simulink model "ScriptDemo"  (R2022b)
settings: configuration reference "TmVcThermal_Configuration_sub" (kept outside this file)
undefined symbols (not defined in the file or in its folder): aaaa, bbbb, cTmComprCtrl_D_u8HvacFlowTable_db, cTmComprCtrl_D_u8HvacFlowTable_sw, cTmComprCtrl_n_i16ChillCmpIMax, cTmComprCtrl_n_i16ChillCmpIMin, cTmComprCtrl_n_i16ChillCmpIMin666, cTmComprCtrl_n_i16ChillCmpPMax, cTmComprCtrl_n_i16ChillCmpPMin, cTmComprCtrl_n_i16CmpChillCoolRpmKiMax, cTmComprCtrl_n_i16CmpChillCoolRpmKiMin, cTmComprCtrl_n_i16CmpChillCoolRpmKpMax, cTmComprCtrl_n_i16CmpChillCoolRpmKpMin, cTmComprCtrl_n_i16CmpCoolRpmKiMax, cTmComprCtrl_n_i16CmpCoolRpmKiMin, cTmComprCtrl_n_i16CmpCoolRpmKpMax, cTmComprCtrl_n_i16CmpCoolRpmKpMin, cTmComprCtrl_n_i16SM4CmpHeatKiMax, cTmComprCtrl_n_i16SM4CmpHeatKiMin, cTmComprCtrl_n_i16SM4CmpHeatKpMax, cTmComprCtrl_n_i16SM4CmpHeatKpMin, cTmComprCtrl_n_i16SM5CmpHeatKiMax, cTmComprCtrl_n_i16SM5CmpHeatKiMin, cTmComprCtrl_n_i16SM5CmpHeatKpMax, cTmComprCtrl_n_i16SM5CmpHeatKpMin, cTmComprCtrl_n_i16SM6CmpHeatKiMax, cTmComprCtrl_n_i16SM6CmpHeatKiMin, cTmComprCtrl_n_i16SM6CmpHeatKpMax, cTmComprCtrl_n_i16SM6CmpHeatKpMin, cTmComprCtrl_n_u16CmpMaxSpdFanFltLimt, cTmComprCtrl_n_u16CmpMaxSpdLoSidePFltLimt, cTmComprCtrl_n_u16CmpMaxSpdSensorFltLimt, cTmComprCtrl_n_u16CompMinRpm, cTmComprCtrl_n_u16CompRpmIncThres, cTmComprCtrl_t_u16BattCooltFFPeriod, cTmComprCtrl_t_u16BattCooltPIPeriod, cTmComprCtrl_t_u16CmpCoolFFPeriod, cTmComprCtrl_t_u16CmpCoolPIPeriod, cTmComprCtrl_t_u16CoolCmpChillFFPeriod, cTmComprCtrl_t_u16CoolCmpChillPIPeriod, cTmComprCtrl_t_u16SM4CmpHeatFFPeriod, cTmComprCtrl_t_u16SM4CmpHeatPIPeriod, cTmComprCtrl_t_u16SM5CmpHeatFFPeriod, cTmComprCtrl_t_u16SM5CmpHeatPIPeriod, cTmComprCtrl_t_u16SM6CmpHeatFFPeriod, cTmComprCtrl_t_u16SM6CmpHeatPIPeriod, cTmComprCtrl_Te_EvapClearInteg, cTmComprCtrl_Te_i16HpReqTempSaturoffset, cTmComprCtrl_Te_i16SatLpReplaceDiff, cTmComprCtrl_Te_i16SM3BatDiffStartEvapDecOffset, cTmComprCtrl_Te_i16SM3EvapLo, cTmComprCtrl_Te_i16SM3TBatDiffEntEvapDecOffset, cTmComprCtrl_Te_i16SM3TBatDiffEntEvapDecOffsetQuit, cTmComprCtrl_Te_s32ErrCmpChillPIContinueCoolH, cTmComprCtrl_Te_s32ErrCmpChillPIContinueCoolL, cTmComprCtrl_Te_s32ErrCmpPIContinueChillH, cTmComprCtrl_Te_s32ErrCmpPIContinueChillL, cTmComprCtrl_Te_s32ErrCmpPIContinueCoolH, cTmComprCtrl_Te_s32ErrCmpPIContinueCoolL, cTmComprCtrl_Te_s32ErrCmpPIContinueHeatH ... (+398)
libraries: simulink x846, PCMULib x711, simulink_need_slupdate x4
(part 10 of 49)

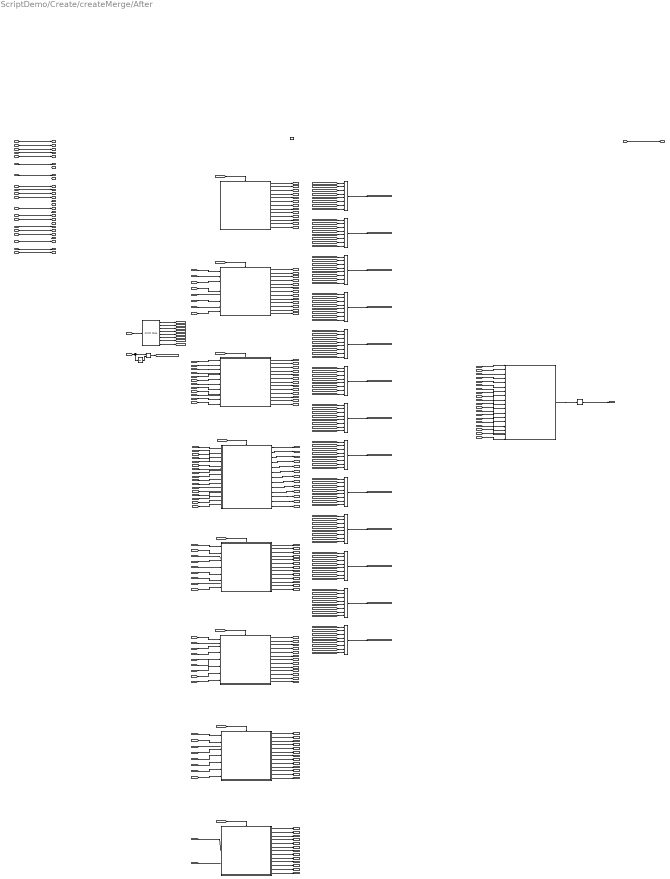
== system ScriptDemo/Create/createMerge/After ==
  note: % 目的: 对当前路径下的，使能子系统或switch case输出的信号，自动生成Merge
      | createMerge( ...
      | 'sigList' , ...
      | { 'rTmComprCtrl_Te_s32LowErrStop' , 'rTmComprCtrl_Te_s32TempError' , ...
      | 'rTmComprCtrl_Te_s32UpErrStop' , 'rTmComprCtrl_n_u16ComprRpmFF' , ...
      | 'rTmComprCtrl_n_u16ComprRpmKi' , 'rTmComprCtrl_n_u16ComprRpmKp' , ...
      | 'rTmComprCtrl_n_u16DisOverrideValue' , 'rTmComprCtrl_n_i16KiLowLimit' , ...
      | 'rTmComprCtrl_n_i16KiUpLimit' , 'rTmComprCtrl_n_i16KpLowLimit' , ...
      | 'rTmComprCtrl_n_i16KpUpLimit' , 'rTmComprCtrl_t_u16PIPeriod' , ...
      | 'xTmComprCtrl_B_Enable' ...
      | }, ...
      | 'resovleSig' ,true)
      |
      | %% 输入参数处理
      | p = inputParser; % 函数的输入解析器
      | addParameter(p, 'sigList' , ...
      | { 'rTmComprCtrl_Te_s32TempError' , 'rTmComprCtrl_n_u16ComprRpmFF' , ...
      | 'rTmComprCtrl_n_u16ComprRpmKp' , 'rTmComprCtrl_n_u16ComprRpmKi' , ...
      | 'rTmComprCtrl_Te_s32UpErrStop' , 'rTmComprCtrl_Te_s32LowErrStop' , ...
      | 'rTmComprCtrl_n_u16KpUpLimit' , 'rTmComprCtrl_n_u16KpLowLimit' , ...
      | 'rTmComprCtrl_n_u16KiUpLimit' , 'rTmComprCtrl_n_u16KiLowLimit' , ...
      | 'rTmComprCtrl_n_u16DisOverrideValue' , 'rTmComprCtrl_t_u8PIPeriod' , ...
      | 'rTmComprCtrl_B_Enable'
      | } ...
      | ); % 设置变量名
      | addParameter(p, 'resovleSig' ,true); % 是否需要解析merge的信号
  sTmComprCtrl_D_u8HvacFlowLevel : Inport  OutDataTypeStr=uint8
  sTmSigProces_Te_s32EvapFanReqRamp : Inport  Port=2  OutDataTypeStr=single
  sTmDiag_D_u8TeEvapFltSt : Inport  Port=3  OutDataTypeStr=uint8
  sTmIn_D_u8DCChrgSt : Inport  Port=4  OutDataTypeStr=uint8
  sTmIn_D_u8HeatPump : Inport  Port=5  OutDataTypeStr=uint8
  sTmIn_Te_s32BattHv : Inport  Port=6  OutDataTypeStr=single
  sTmIn_X_s32ClimtRcirc : Inport  Port=7  OutDataTypeStr=single
  sTmSigProces_D_u8BattThermReq : Inport  Port=8  OutDataTypeStr=uint8
  sTmSigProces_D_u8HvBattCoolgReq : Inport  Port=9  OutDataTypeStr=uint8
  sTmSigProces_Te_s32EvapFanFilter : Inport  Port=10  OutDataTypeStr=single
  sTmSigProces_Te_s32HeatrAirTReqRamp : Inport  Port=11  OutDataTypeStr=single
  sTmSigProces_Te_s32HvacHexAirTFilter : Inport  Port=12  OutDataTypeStr=single
  sTmSigProces_Te_s32SatHp : Inport  Port=13  OutDataTypeStr=single
  sTmSigProces_Te_s32SatLp : Inport  Port=14  OutDataTypeStr=single
  xTmComprCtrl_B_CompOnReqCompOn : Inport  Port=15  OutDataTypeStr=boolean
  xTmComprCtrl_B_ReduceRpm : Inport  Port=16  OutDataTypeStr=boolean
  yTmHvchCtrl_B_HpcPtcEnad : Inport  Port=17  OutDataTypeStr=boolean
  yTmRefriModeMgr_B_CoolOCRMode : Inport  Port=18  OutDataTypeStr=boolean
  sTmSigProces_Pw_i16ReqPwrForCool : Inport  Port=19  OutDataTypeStr=int16
  yTmRefriModeMgr_B_HeatModeInCycle : Inport  Port=20  OutDataTypeStr=boolean
  Enable : EnablePort
  ID29332_RpmPI : Subsystem
  Merge{,1..12} (13 alike) : Merge  Inputs=8
  Relational Operator : RelationalOperator  Operator=~=  OutDataTypeStr=boolean  RndMeth=Simplest  InputSameDT=off
  SM0 : Subsystem
  SM1SM21 : Subsystem
  SM2SM22 : Subsystem
  SM3SM23 : Subsystem
  SM4 : Subsystem
  SM5 : Subsystem
  SM6 : Subsystem
  SM7 : Subsystem
  Signal Conversion : SignalConversion  OverrideOpt=off
  Switch Case : SwitchCase  CaseConditions={0,[1,21],[2,22],[3,23],4,5,6,7}  ShowDefaultCase=off
  Unit Delay : UnitDelay  SampleTime=-1  HasFrameUpgradeWarning=on
  sTmComprCtrl_n_u16CompRpmReqNorm : Outport  OutDataTypeStr=uint16
  wires:
  [yTmRefriModeMgr_B_CoolOCRMode] -> SM2SM22/9(yTmRefriModeMgr_B_CoolOCRMode)
  ? -> [sTmIn_Te_s32HvBattCooltTReq]
  [sTmSigProces_D_u8BattThermReq] -> SM3SM23/8(sTmSigProces_D_u8BattThermReq)
  [sTmSigProces_Te_s32TempInlet] -> ?
  ? -> [yTmRefriModeMgr_B_CoolModeInCycle]
  [sTmSigProces_Te_s32SatHp] -> SM5/4(sTmSigProces_Te_s32SatHp)
  [sTmRefriModeMgr_D_u8HPCurMode] -> ?
  [yTmRefriModeMgr_B_HeatModeInCycle] -> SM4/7(yTmRefriModeMgr_B_HeatModeInCycle)
  [xTmComprCtrl_B_ModeChanged] -> SM3SM23/13(xTmComprCtrl_B_ModeChanged)
  [yTmRefriModeMgr_B_HeatModeInCycle] -> SM6/7(yTmRefriModeMgr_B_HeatModeInCycle)
  [yTmRefriModeMgr_B_CoolModeInCycle] -> ?
  [SM5] -> SM5/Action
  sTmSigProces_Te_s32SatLp/1 -> [sTmSigProces_Te_s32SatLp]
  sTmIn_X_s32ClimtRcirc/1 -> [sTmIn_X_s32ClimtRcirc]
  yTmRefriModeMgr_B_HeatModeInCycle/1 -> [yTmRefriModeMgr_B_HeatModeInCycle]
  yTmRefriModeMgr_B_CoolOCRMode/1 -> [yTmRefriModeMgr_B_CoolOCRMode]
  [yTmRefriModeMgr_B_HeatModeInCycle] -> ID29332_RpmPI/18(yTmRefriModeMgr_B_HeatModeInCycle)
  yTmHvchCtrl_B_HpcPtcEnad/1 -> [yTmHvchCtrl_B_HpcPtcEnad]
  [sTmSigProces_Te_s32EvapFanFilter] -> ID29332_RpmPI/17(sTmSigProces_Te_s32EvapFanFilter)
  [sTmSigProces_D_u8HvBattCoolgReq] -> SM3SM23/9(sTmSigProces_D_u8HvBattCoolgReq)
  [sTmSigProces_Te_s32HvacHexAirTFilter] -> SM5/3(sTmSigProces_Te_s32HvacHexAirTFilter)
  ? -> [sTmSigProces_Te_s32HvBattCooltTFilter]
  [yTmRefriModeMgr_B_CoolOCRMode] -> SM3SM23/14(yTmRefriModeMgr_B_CoolOCRMode)
  [yTmHvchCtrl_B_HpcPtcEnad] -> SM5/7(yTmHvchCtrl_B_HpcPtcEnad)
  [sTmComprCtrl_D_u8HvacFlowLevel] -> SM5/5(sTmComprCtrl_D_u8HvacFlowLevel)
  sTmSigProces_D_u8HvBattCoolgReq/1 -> [sTmSigProces_D_u8HvBattCoolgReq]
  [xTmComprCtrl_B_ReduceRpm] -> ID29332_RpmPI/16(xTmComprCtrl_B_ReduceRpm)
  ? -> [sTmSigProces_Te_s32HvBattCooltTOutFilter]
  sTmSigProces_Pw_i16ReqPwrForCool/1 -> [sTmSigProces_Pw_i16ReqPwrForCool]
  [sTmSigProces_Te_s32TAmb] -> ?
  [sTmIn_Te_s32BattHv] -> SM3SM23/5(sTmIn_Te_s32BattHv)
  [sTmComprCtrl_D_u8HvacFlowLevel] -> SM6/4(sTmComprCtrl_D_u8HvacFlowLevel)
  Switch Case/7 -> [SM6]
  Switch Case/5 -> [SM4]
  ? -> [sTmSigProces_Te_s32TempInlet]
  [xTmComprCtrl_B_CompOnReqCompOn] -> SM5/6(xTmComprCtrl_B_CompOnReqCompOn)
  [rTmComprCtrl_n_u16ComprRpmKp] -> ID29332_RpmPI/6(rTmComprCtrl_n_u16ComprRpmKp)
  [SM0] -> SM0/Action
  xTmComprCtrl_B_ReduceRpm/1 -> [xTmComprCtrl_B_ReduceRpm]
  [sTmSigProces_Te_s32HeatrAirTReqRamp] -> SM6/1(sTmSigProces_Te_s32HeatrAirTReqRamp)
  Relational Operator/1 -> [xTmComprCtrl_B_ModeChanged]
  [xTmComprCtrl_B_CompOnReqCompOn] -> SM3SM23/12(xTmComprCtrl_B_CompOnReqCompOn)
  sTmSigProces_Te_s32EvapFanFilter/1 -> [sTmSigProces_Te_s32EvapFanFilter]
  [xTmComprCtrl_B_CompOnReqCompOn] -> SM6/5(xTmComprCtrl_B_CompOnReqCompOn)
  [sTmSigProces_Te_s32HvacHexAirTFilter] -> SM4/2(sTmSigProces_Te_s32HvacHexAirTFilter)
  [sTmSigProces_Te_s32HvBattCooltTFilter] -> ?
  [yTmHvchCtrl_B_HpcPtcEnad] -> SM6/6(yTmHvchCtrl_B_HpcPtcEnad)
  [rTmComprCtrl_Te_s32TempError] -> ID29332_RpmPI/2(rTmComprCtrl_Te_s32TempError)
  [sTmSigProces_Te_s32SatHp] -> SM6/3(sTmSigProces_Te_s32SatHp)
  [sTmIn_D_u8DCChrgSt] -> SM1SM21/1(sTmIn_D_u8DCChrgSt)
  [SM6] -> SM6/Action
  [sTmIn_D_u8DCChrgSt] -> SM3SM23/3(sTmIn_D_u8DCChrgSt)
  [xTmComprCtrl_B_CompOnReqCompOn] -> SM4/5(xTmComprCtrl_B_CompOnReqCompOn)
  [sTmSigProces_Te_s32HvBattCooltTFilter] -> ?
  Switch Case/4 -> [SM3_SM23]
  [rTmComprCtrl_n_u16ComprRpmFF] -> ID29332_RpmPI/4(rTmComprCtrl_n_u16ComprRpmFF)
  [xTmComprCtrl_B_Enable] -> ID29332_RpmPI/14(xTmComprCtrl_B_Enable)
  [sTmSigProces_Te_s32TAmb] -> ?
  [rTmComprCtrl_n_i16KpLowLimit] -> ID29332_RpmPI/10(rTmComprCtrl_n_i16KpLowLimit)
  [rTmComprCtrl_n_u16DisOverrideValue] -> ID29332_RpmPI/7(rTmComprCtrl_n_u16DisOverrideValue)
  xTmComprCtrl_B_CompOnReqCompOn/1 -> [xTmComprCtrl_B_CompOnReqCompOn]
  [rTmComprCtrl_n_u16ComprRpmKi] -> ID29332_RpmPI/5(rTmComprCtrl_n_u16ComprRpmKi)
  [rTmComprCtrl_n_i16KiLowLimit] -> ID29332_RpmPI/8(rTmComprCtrl_n_i16KiLowLimit)
  [xTmComprCtrl_B_ModeChanged] -> ID29332_RpmPI/15(xTmComprCtrl_B_ModeChanged)
  [sTmSigProces_Te_s32HvBattCooltTFilter] -> ?
  [sTmSigProces_Te_s32TempInlet] -> ?
  [sTmIn_Te_s32HvBattCooltTReq] -> ?
  Unit Delay/1 -> Relational Operator/2
  [SM2_SM22] -> SM2SM22/Action
  [sTmIn_D_u8HeatPump] -> SM3SM23/4(sTmIn_D_u8HeatPump)
  [sTmSigProces_Te_s32TAmb] -> ?
  [sTmRefriModeMgr_D_u8HPCurMode] -> Switch Case/1
  [sTmSigProces_Te_s32HeatrAirTReqRamp] -> SM5/2(sTmSigProces_Te_s32HeatrAirTReqRamp)
  [rTmComprCtrl_n_i16KpUpLimit] -> ID29332_RpmPI/11(rTmComprCtrl_n_i16KpUpLimit)
  [sTmComprCtrl_D_u8HvacFlowLevel] -> SM3SM23/7(sTmComprCtrl_D_u8HvacFlowLevel)
  [rTmComprCtrl_Te_s32LowErrStop] -> ID29332_RpmPI/1(rTmComprCtrl_Te_s32LowErrStop)
  [sTmSigProces_Te_s32EvapFanReqRamp] -> SM3SM23/1(sTmSigProces_Te_s32EvapFanReqRamp)
  [sTmSigProces_D_u8HvBattCoolgReq] -> SM1SM21/3(sTmSigProces_D_u8HvBattCoolgReq)
  [sTmComprCtrl_D_u8HvacFlowLevel] -> SM2SM22/5(sTmComprCtrl_D_u8HvacFlowLevel)
  Switch Case/8 -> [SM7]
  [sTmSigProces_Te_s32EvapFanReqRamp] -> SM2SM22/1(sTmSigProces_Te_s32EvapFanReqRamp)
  [sTmRefriModeMgr_D_u8HPCurMode] -> Unit Delay/1, Relational Operator/1
  [SM4] -> SM4/Action
  [sTmSigProces_Te_s32SatLp] -> SM2SM22/7(sTmSigProces_Te_s32SatLp)
  [sTmIn_D_u8HeatPump] -> SM2SM22/3(sTmIn_D_u8HeatPump)
  [sTmSigProces_Te_s32SatLp] -> SM3SM23/11(sTmSigProces_Te_s32SatLp)
  [sTmSigProces_Te_s32EvapFanFilter] -> SM2SM22/6(sTmSigProces_Te_s32EvapFanFilter)
  [sTmSigProces_Te_s32SatHp] -> SM4/3(sTmSigProces_Te_s32SatHp)
  [sTmSigProces_Pw_i16ReqPwrForCool] -> SM2SM22/10(sTmSigProces_Pw_i16ReqPwrForCool)
  [SM7] -> SM7/Action
  ? -> [sTmSigProces_Te_s32TAmb]
  [sTmSigProces_Te_s32TempInlet] -> ?
  [sTmDiag_D_u8TeEvapFltSt] -> SM3SM23/2(sTmDiag_D_u8TeEvapFltSt)
  [sTmSigProces_Te_s32HvacHexAirTFilter] -> SM6/2(sTmSigProces_Te_s32HvacHexAirTFilter)
  [sTmSigProces_Te_s32TAmb] -> ?
  [sTmIn_D_u8HeatPump] -> SM1SM21/5(sTmIn_D_u8HeatPump)
  [yTmRefriModeMgr_B_CoolModeInCycle] -> ?
  [sTmIn_X_s32ClimtRcirc] -> SM2SM22/4(sTmIn_X_s32ClimtRcirc)
  [SM1_SM21] -> SM1SM21/Action
  [sTmIn_X_s32ClimtRcirc] -> SM3SM23/6(sTmIn_X_s32ClimtRcirc)
  [sRpmPI_n_u16CompRpmReq] -> sTmComprCtrl_n_u16CompRpmReqNorm/1
  [sTmSigProces_Te_s32EvapFanFilter] -> SM3SM23/10(sTmSigProces_Te_s32EvapFanFilter)
  Signal Conversion/1 -> [sRpmPI_n_u16CompRpmReq]
  [sTmSigProces_Te_s32TAmb] -> ?
  [sTmDiag_D_u8TeEvapFltSt] -> SM2SM22/2(sTmDiag_D_u8TeEvapFltSt)
  sTmSigProces_Te_s32HeatrAirTReqRamp/1 -> [sTmSigProces_Te_s32HeatrAirTReqRamp]
  [xTmComprCtrl_B_CompOnReqCompOn] -> ID29332_RpmPI/13(xTmComprCtrl_B_CompOnReqCompOn)
  sTmComprCtrl_D_u8HvacFlowLevel/1 -> [sTmComprCtrl_D_u8HvacFlowLevel]
  [sTmSigProces_Te_s32HvBattCooltTOutFilter] -> ?
  sTmDiag_D_u8TeEvapFltSt/1 -> [sTmDiag_D_u8TeEvapFltSt]
  sTmSigProces_Te_s32SatHp/1 -> [sTmSigProces_Te_s32SatHp]
  ? -> [sTmRefriModeMgr_D_u8HPCurMode]
  [xTmComprCtrl_B_CompOnReqCompOn] -> SM1SM21/4(xTmComprCtrl_B_CompOnReqCompOn)
  sTmIn_D_u8DCChrgSt/1 -> [sTmIn_D_u8DCChrgSt]
  [yTmHvchCtrl_B_HpcPtcEnad] -> SM4/6(yTmHvchCtrl_B_HpcPtcEnad)
  [sTmComprCtrl_D_u8HvacFlowLevel] -> SM4/4(sTmComprCtrl_D_u8HvacFlowLevel)
  [sTmIn_Te_s32HvBattCooltTReq] -> ?
  sTmSigProces_Te_s32EvapFanReqRamp/1 -> [sTmSigProces_Te_s32EvapFanReqRamp]
  Switch Case/6 -> [SM5]
  sTmSigProces_Te_s32HvacHexAirTFilter/1 -> [sTmSigProces_Te_s32HvacHexAirTFilter]
  [sTmSigProces_Te_s32SatLp] -> SM5/1(sTmSigProces_Te_s32SatLp)
  Switch Case/3 -> [SM2_SM22]
  ID29332_RpmPI/1(rTmComprCtrl_n_u16CompRpmReqPI) -> Signal Conversion/1  "rTmComprCtrl_n_u16CompRpmReqPI"
  [sTmSigProces_Te_s32HeatrAirTReqRamp] -> SM4/1(sTmSigProces_Te_s32HeatrAirTReqRamp)
  [SM3_SM23] -> SM3SM23/Action
  sTmIn_D_u8HeatPump/1 -> [sTmIn_D_u8HeatPump]
  sTmSigProces_D_u8BattThermReq/1 -> [sTmSigProces_D_u8BattThermReq]
  [rTmComprCtrl_t_u16PIPeriod] -> ID29332_RpmPI/12(rTmComprCtrl_t_u16PIPeriod)
  [sTmSigProces_D_u8BattThermReq] -> SM1SM21/2(sTmSigProces_D_u8BattThermReq)
  Switch Case/2 -> [SM1_SM21]
  Switch Case/1 -> [SM0]
  [rTmComprCtrl_Te_s32UpErrStop] -> ID29332_RpmPI/3(rTmComprCtrl_Te_s32UpErrStop)
  [xTmComprCtrl_B_CompOnReqCompOn] -> SM2SM22/8(xTmComprCtrl_B_CompOnReqCompOn)
  sTmIn_Te_s32BattHv/1 -> [sTmIn_Te_s32BattHv]
  [rTmComprCtrl_n_i16KiUpLimit] -> ID29332_RpmPI/9(rTmComprCtrl_n_i16KiUpLimit)
  SM7/1(rSM7_n_u16DisOverrideValue) -> [rSM7_n_u16DisOverrideValue]
  SM7/2(rSM7_t_u16PIPeriod) -> [rSM7_t_u16PIPeriod]
  SM7/3(xSM7_B_Enable) -> [xSM7_B_Enable]
  SM7/4(rSM7_n_i16KiUpLimit) -> [rSM7_n_i16KiUpLimit]
  SM7/5(rSM7_n_i16KiLowLimit) -> [rSM7_n_i16KiLowLimit]
  SM7/6(rSM7_Te_s32TempError) -> [rSM7_Te_s32TempError]
  SM7/7(rSM7_n_u16ComprRpmFF) -> [rSM7_n_u16ComprRpmFF]
  SM7/8(rSM7_n_u16ComprRpmKp) -> [rSM7_n_u16ComprRpmKp]
  SM7/9(rSM7_n_u16ComprRpmKi) -> [rSM7_n_u16ComprRpmKi]
  SM7/10(rSM7_Te_s32UpErrStop) -> [rSM7_Te_s32UpErrStop]
  SM7/11(rSM7_Te_s32LowErrStop) -> [rSM7_Te_s32LowErrStop]
  SM7/12(rSM7_n_i16KpUpLimit) -> [rSM7_n_i16KpUpLimit]
  SM7/13(rSM7_n_i16KpLowLimit) -> [rSM7_n_i16KpLowLimit]
  SM3SM23/1(rSM3SM23_n_u16ComprRpmKi) -> [rSM3SM23_n_u16ComprRpmKi]
  SM3SM23/2(rSM3SM23_Te_s32UpErrStop) -> [rSM3SM23_Te_s32UpErrStop]
  SM3SM23/3(rSM3SM23_n_u16ComprRpmFF) -> [rSM3SM23_n_u16ComprRpmFF]
  SM3SM23/4(rSM3SM23_n_u16DisOverrideValue) -> [rSM3SM23_n_u16DisOverrideValue]
  SM3SM23/5(rSM3SM23_t_u16PIPeriod) -> [rSM3SM23_t_u16PIPeriod]
  SM3SM23/6(xSM3SM23_B_Enable) -> [xSM3SM23_B_Enable]
  SM3SM23/7(rSM3SM23_n_u16ComprRpmKp) -> [rSM3SM23_n_u16ComprRpmKp]
  SM3SM23/8(rSM3SM23_Te_s32LowErrStop) -> [rSM3SM23_Te_s32LowErrStop]
  SM3SM23/9(rSM3SM23_n_i16KpUpLimit) -> [rSM3SM23_n_i16KpUpLimit]
  SM3SM23/10(rSM3SM23_n_i16KpLowLimit) -> [rSM3SM23_n_i16KpLowLimit]
  SM3SM23/11(rSM3SM23_n_i16KiUpLimit) -> [rSM3SM23_n_i16KiUpLimit]
  SM3SM23/12(rSM3SM23_n_i16KiLowLimit) -> [rSM3SM23_n_i16KiLowLimit]
  SM3SM23/13(rSM3SM23_Te_s32TempError) -> [rSM3SM23_Te_s32TempError]
  SM0/1(rSM0_Te_s32TempError) -> [rSM0_Te_s32TempError]
  SM0/2(rSM0_n_u16ComprRpmFF) -> [rSM0_n_u16ComprRpmFF]
  SM0/3(rSM0_n_u16DisOverrideValue) -> [rSM0_n_u16DisOverrideValue]
  SM0/4(rSM0_t_u16PIPeriod) -> [rSM0_t_u16PIPeriod]
  SM0/5(xSM0_B_Enable) -> [xSM0_B_Enable]
  SM0/6(rSM0_n_u16ComprRpmKp) -> [rSM0_n_u16ComprRpmKp]
  SM0/7(rSM0_n_u16ComprRpmKi) -> [rSM0_n_u16ComprRpmKi]
  SM0/8(rSM0_Te_s32UpErrStop) -> [rSM0_Te_s32UpErrStop]
  SM0/9(rSM0_Te_s32LowErrStop) -> [rSM0_Te_s32LowErrStop]
  SM0/10(rSM0_n_i16KpUpLimit) -> [rSM0_n_i16KpUpLimit]
  SM0/11(rSM0_n_i16KpLowLimit) -> [rSM0_n_i16KpLowLimit]
  SM0/12(rSM0_n_i16KiUpLimit) -> [rSM0_n_i16KiUpLimit]
  SM0/13(rSM0_n_i16KiLowLimit) -> [rSM0_n_i16KiLowLimit]
  SM1SM21/1(rSM1SM21_n_u16DisOverrideValue) -> [rSM1SM21_n_u16DisOverrideValue]
  SM1SM21/2(rSM1SM21_t_u16PIPeriod) -> [rSM1SM21_t_u16PIPeriod]
  SM1SM21/3(rSM1SM21_Te_s32UpErrStop) -> [rSM1SM21_Te_s32UpErrStop]
  SM1SM21/4(rSM1SM21_Te_s32LowErrStop) -> [rSM1SM21_Te_s32LowErrStop]
  SM1SM21/5(rSM1SM21_n_i16KpUpLimit) -> [rSM1SM21_n_i16KpUpLimit]
  SM1SM21/6(rSM1SM21_n_u16ComprRpmFF) -> [rSM1SM21_n_u16ComprRpmFF]
  SM1SM21/7(rSM1SM21_n_u16ComprRpmKp) -> [rSM1SM21_n_u16ComprRpmKp]
  SM1SM21/8(rSM1SM21_n_u16ComprRpmKi) -> [rSM1SM21_n_u16ComprRpmKi]
  SM1SM21/9(rSM1SM21_n_i16KpLowLimit) -> [rSM1SM21_n_i16KpLowLimit]
  SM1SM21/10(rSM1SM21_n_i16KiUpLimit) -> [rSM1SM21_n_i16KiUpLimit]
  SM1SM21/11(rSM1SM21_n_i16KiLowLimit) -> [rSM1SM21_n_i16KiLowLimit]
  SM1SM21/12(xSM1SM21_B_Enable) -> [xSM1SM21_B_Enable]
  SM1SM21/13(rSM1SM21_Te_s32TempError) -> [rSM1SM21_Te_s32TempError]
  SM2SM22/1(rSM2SM22_n_u16DisOverrideValue) -> [rSM2SM22_n_u16DisOverrideValue]
  SM2SM22/2(rSM2SM22_t_u16PIPeriod) -> [rSM2SM22_t_u16PIPeriod]
  SM2SM22/3(rSM2SM22_Te_s32UpErrStop) -> [rSM2SM22_Te_s32UpErrStop]
  SM2SM22/4(rSM2SM22_n_u16ComprRpmFF) -> [rSM2SM22_n_u16ComprRpmFF]
  SM2SM22/5(rSM2SM22_n_u16ComprRpmKp) -> [rSM2SM22_n_u16ComprRpmKp]
  SM2SM22/6(rSM2SM22_n_u16ComprRpmKi) -> [rSM2SM22_n_u16ComprRpmKi]
  SM2SM22/7(rSM2SM22_Te_s32LowErrStop) -> [rSM2SM22_Te_s32LowErrStop]
  SM2SM22/8(rSM2SM22_n_i16KpUpLimit) -> [rSM2SM22_n_i16KpUpLimit]
  SM2SM22/9(rSM2SM22_n_i16KpLowLimit) -> [rSM2SM22_n_i16KpLowLimit]
  SM2SM22/10(rSM2SM22_n_i16KiUpLimit) -> [rSM2SM22_n_i16KiUpLimit]
  SM2SM22/11(rSM2SM22_n_i16KiLowLimit) -> [rSM2SM22_n_i16KiLowLimit]
  SM2SM22/12(xSM2SM22_B_Enable) -> [xSM2SM22_B_Enable]
  SM2SM22/13(rSM2SM22_Te_s32TempError) -> [rSM2SM22_Te_s32TempError]
  SM4/1(rSM4_n_u16DisOverrideValue) -> [rSM4_n_u16DisOverrideValue]
  SM4/2(rSM4_t_u16PIPeriod) -> [rSM4_t_u16PIPeriod]
  SM4/3(rSM4_Te_s32UpErrStop) -> [rSM4_Te_s32UpErrStop]
  SM4/4(rSM4_n_u16ComprRpmFF) -> [rSM4_n_u16ComprRpmFF]
  SM4/5(rSM4_n_u16ComprRpmKp) -> [rSM4_n_u16ComprRpmKp]
  SM4/6(rSM4_Te_s32LowErrStop) -> [rSM4_Te_s32LowErrStop]
  SM4/7(rSM4_n_i16KpUpLimit) -> [rSM4_n_i16KpUpLimit]
  SM4/8(rSM4_n_i16KpLowLimit) -> [rSM4_n_i16KpLowLimit]
  SM4/9(rSM4_n_i16KiUpLimit) -> [rSM4_n_i16KiUpLimit]
  SM4/10(rSM4_n_i16KiLowLimit) -> [rSM4_n_i16KiLowLimit]
  SM4/11(xSM4_B_Enable) -> [xSM4_B_Enable]
  SM4/12(rSM4_n_u16ComprRpmKi) -> [rSM4_n_u16ComprRpmKi]
  SM4/13(rSM4_Te_s32TempError) -> [rSM4_Te_s32TempError]
  SM5/1(rSM5_n_u16DisOverrideValue) -> [rSM5_n_u16DisOverrideValue]
  SM5/2(rSM5_t_u16PIPeriod) -> [rSM5_t_u16PIPeriod]
  SM5/3(rSM5_Te_s32UpErrStop) -> [rSM5_Te_s32UpErrStop]
  SM5/4(rSM5_n_u16ComprRpmFF) -> [rSM5_n_u16ComprRpmFF]
  SM5/5(rSM5_n_u16ComprRpmKp) -> [rSM5_n_u16ComprRpmKp]
  SM5/6(rSM5_Te_s32LowErrStop) -> [rSM5_Te_s32LowErrStop]
  SM5/7(rSM5_n_i16KpUpLimit) -> [rSM5_n_i16KpUpLimit]
  SM5/8(rSM5_n_i16KpLowLimit) -> [rSM5_n_i16KpLowLimit]
  SM5/9(rSM5_n_i16KiUpLimit) -> [rSM5_n_i16KiUpLimit]
  SM5/10(rSM5_n_i16KiLowLimit) -> [rSM5_n_i16KiLowLimit]
  SM5/11(xSM5_B_Enable) -> [xSM5_B_Enable]
  SM5/12(rSM5_n_u16ComprRpmKi) -> [rSM5_n_u16ComprRpmKi]
  SM5/13(rSM5_Te_s32TempError) -> [rSM5_Te_s32TempError]
  SM6/1(rSM6_n_u16DisOverrideValue) -> [rSM6_n_u16DisOverrideValue]
  SM6/2(rSM6_t_u16PIPeriod) -> [rSM6_t_u16PIPeriod]
  SM6/3(rSM6_Te_s32UpErrStop) -> [rSM6_Te_s32UpErrStop]
  SM6/4(rSM6_n_u16ComprRpmFF) -> [rSM6_n_u16ComprRpmFF]
  SM6/5(rSM6_n_u16ComprRpmKp) -> [rSM6_n_u16ComprRpmKp]
  SM6/6(rSM6_Te_s32LowErrStop) -> [rSM6_Te_s32LowErrStop]
  SM6/7(rSM6_n_i16KpUpLimit) -> [rSM6_n_i16KpUpLimit]
  SM6/8(rSM6_n_i16KpLowLimit) -> [rSM6_n_i16KpLowLimit]
  SM6/9(rSM6_n_i16KiUpLimit) -> [rSM6_n_i16KiUpLimit]
  SM6/10(rSM6_n_i16KiLowLimit) -> [rSM6_n_i16KiLowLimit]
  SM6/11(xSM6_B_Enable) -> [xSM6_B_Enable]
  SM6/12(rSM6_n_u16ComprRpmKi) -> [rSM6_n_u16ComprRpmKi]
  SM6/13(rSM6_Te_s32TempError) -> [rSM6_Te_s32TempError]
  [rSM0_Te_s32LowErrStop] -> Merge/1
  [rSM1SM21_Te_s32LowErrStop] -> Merge/2
  [rSM2SM22_Te_s32LowErrStop] -> Merge/3
  [rSM3SM23_Te_s32LowErrStop] -> Merge/4
  [rSM4_Te_s32LowErrStop] -> Merge/5
  [rSM5_Te_s32LowErrStop] -> Merge/6
  [rSM6_Te_s32LowErrStop] -> Merge/7
  [rSM7_Te_s32LowErrStop] -> Merge/8
  Merge/1 -> [rTmComprCtrl_Te_s32LowErrStop]  "rTmComprCtrl_Te_s32LowErrStop"
  [rSM0_Te_s32TempError] -> Merge1/1
  [rSM1SM21_Te_s32TempError] -> Merge1/2
  [rSM2SM22_Te_s32TempError] -> Merge1/3
  [rSM3SM23_Te_s32TempError] -> Merge1/4
  [rSM4_Te_s32TempError] -> Merge1/5
  [rSM5_Te_s32TempError] -> Merge1/6
  [rSM6_Te_s32TempError] -> Merge1/7
  [rSM7_Te_s32TempError] -> Merge1/8
  Merge1/1 -> [rTmComprCtrl_Te_s32TempError]  "rTmComprCtrl_Te_s32TempError"
  [rSM0_Te_s32UpErrStop] -> Merge2/1
  [rSM1SM21_Te_s32UpErrStop] -> Merge2/2
  [rSM2SM22_Te_s32UpErrStop] -> Merge2/3
  [rSM3SM23_Te_s32UpErrStop] -> Merge2/4
  [rSM4_Te_s32UpErrStop] -> Merge2/5
  [rSM5_Te_s32UpErrStop] -> Merge2/6
  [rSM6_Te_s32UpErrStop] -> Merge2/7
  [rSM7_Te_s32UpErrStop] -> Merge2/8
  Merge2/1 -> [rTmComprCtrl_Te_s32UpErrStop]  "rTmComprCtrl_Te_s32UpErrStop"
  [rSM0_n_u16ComprRpmFF] -> Merge3/1
  [rSM1SM21_n_u16ComprRpmFF] -> Merge3/2
  [rSM2SM22_n_u16ComprRpmFF] -> Merge3/3
  [rSM3SM23_n_u16ComprRpmFF] -> Merge3/4
  [rSM4_n_u16ComprRpmFF] -> Merge3/5
  [rSM5_n_u16ComprRpmFF] -> Merge3/6
  [rSM6_n_u16ComprRpmFF] -> Merge3/7
  [rSM7_n_u16ComprRpmFF] -> Merge3/8
  Merge3/1 -> [rTmComprCtrl_n_u16ComprRpmFF]  "rTmComprCtrl_n_u16ComprRpmFF"
  [rSM0_n_u16ComprRpmKi] -> Merge4/1
  [rSM1SM21_n_u16ComprRpmKi] -> Merge4/2
  [rSM2SM22_n_u16ComprRpmKi] -> Merge4/3
  [rSM3SM23_n_u16ComprRpmKi] -> Merge4/4
  [rSM4_n_u16ComprRpmKi] -> Merge4/5
  [rSM5_n_u16ComprRpmKi] -> Merge4/6
  [rSM6_n_u16ComprRpmKi] -> Merge4/7
  [rSM7_n_u16ComprRpmKi] -> Merge4/8
  Merge4/1 -> [rTmComprCtrl_n_u16ComprRpmKi]  "rTmComprCtrl_n_u16ComprRpmKi"
  [rSM0_n_u16ComprRpmKp] -> Merge5/1
  [rSM1SM21_n_u16ComprRpmKp] -> Merge5/2
  [rSM2SM22_n_u16ComprRpmKp] -> Merge5/3
  [rSM3SM23_n_u16ComprRpmKp] -> Merge5/4
  [rSM4_n_u16ComprRpmKp] -> Merge5/5
  [rSM5_n_u16ComprRpmKp] -> Merge5/6
  [rSM6_n_u16ComprRpmKp] -> Merge5/7
  [rSM7_n_u16ComprRpmKp] -> Merge5/8
  Merge5/1 -> [rTmComprCtrl_n_u16ComprRpmKp]  "rTmComprCtrl_n_u16ComprRpmKp"
  [rSM0_n_u16DisOverrideValue] -> Merge6/1
  [rSM1SM21_n_u16DisOverrideValue] -> Merge6/2
  [rSM2SM22_n_u16DisOverrideValue] -> Merge6/3
  [rSM3SM23_n_u16DisOverrideValue] -> Merge6/4
  [rSM4_n_u16DisOverrideValue] -> Merge6/5
  [rSM5_n_u16DisOverrideValue] -> Merge6/6
  [rSM6_n_u16DisOverrideValue] -> Merge6/7
  [rSM7_n_u16DisOverrideValue] -> Merge6/8
  Merge6/1 -> [rTmComprCtrl_n_u16DisOverrideValue]  "rTmComprCtrl_n_u16DisOverrideValue"
  [rSM0_n_i16KiLowLimit] -> Merge7/1
  [rSM1SM21_n_i16KiLowLimit] -> Merge7/2
  [rSM2SM22_n_i16KiLowLimit] -> Merge7/3
  [rSM3SM23_n_i16KiLowLimit] -> Merge7/4
  [rSM4_n_i16KiLowLimit] -> Merge7/5
  [rSM5_n_i16KiLowLimit] -> Merge7/6
  [rSM6_n_i16KiLowLimit] -> Merge7/7
  [rSM7_n_i16KiLowLimit] -> Merge7/8
  Merge7/1 -> [rTmComprCtrl_n_i16KiLowLimit]  "rTmComprCtrl_n_i16KiLowLimit"
  [rSM0_n_i16KiUpLimit] -> Merge8/1
  [rSM1SM21_n_i16KiUpLimit] -> Merge8/2
  [rSM2SM22_n_i16KiUpLimit] -> Merge8/3
  [rSM3SM23_n_i16KiUpLimit] -> Merge8/4
  [rSM4_n_i16KiUpLimit] -> Merge8/5
  [rSM5_n_i16KiUpLimit] -> Merge8/6
  [rSM6_n_i16KiUpLimit] -> Merge8/7
  [rSM7_n_i16KiUpLimit] -> Merge8/8
  Merge8/1 -> [rTmComprCtrl_n_i16KiUpLimit]  "rTmComprCtrl_n_i16KiUpLimit"
  [rSM0_n_i16KpLowLimit] -> Merge9/1
  [rSM1SM21_n_i16KpLowLimit] -> Merge9/2
  [rSM2SM22_n_i16KpLowLimit] -> Merge9/3
  [rSM3SM23_n_i16KpLowLimit] -> Merge9/4
  [rSM4_n_i16KpLowLimit] -> Merge9/5
  [rSM5_n_i16KpLowLimit] -> Merge9/6
  [rSM6_n_i16KpLowLimit] -> Merge9/7
  [rSM7_n_i16KpLowLimit] -> Merge9/8
  Merge9/1 -> [rTmComprCtrl_n_i16KpLowLimit]  "rTmComprCtrl_n_i16KpLowLimit"
  [rSM0_n_i16KpUpLimit] -> Merge10/1
  [rSM1SM21_n_i16KpUpLimit] -> Merge10/2
  [rSM2SM22_n_i16KpUpLimit] -> Merge10/3
  [rSM3SM23_n_i16KpUpLimit] -> Merge10/4
  [rSM4_n_i16KpUpLimit] -> Merge10/5
  [rSM5_n_i16KpUpLimit] -> Merge10/6
  [rSM6_n_i16KpUpLimit] -> Merge10/7
  [rSM7_n_i16KpUpLimit] -> Merge10/8
  Merge10/1 -> [rTmComprCtrl_n_i16KpUpLimit]  "rTmComprCtrl_n_i16KpUpLimit"
  [rSM0_t_u16PIPeriod] -> Merge11/1
  [rSM1SM21_t_u16PIPeriod] -> Merge11/2
  [rSM2SM22_t_u16PIPeriod] -> Merge11/3
  [rSM3SM23_t_u16PIPeriod] -> Merge11/4
  [rSM4_t_u16PIPeriod] -> Merge11/5
  [rSM5_t_u16PIPeriod] -> Merge11/6
  [rSM6_t_u16PIPeriod] -> Merge11/7
  [rSM7_t_u16PIPeriod] -> Merge11/8
  Merge11/1 -> [rTmComprCtrl_t_u16PIPeriod]  "rTmComprCtrl_t_u16PIPeriod"
  [xSM0_B_Enable] -> Merge12/1
  [xSM1SM21_B_Enable] -> Merge12/2
  [xSM2SM22_B_Enable] -> Merge12/3
  [xSM3SM23_B_Enable] -> Merge12/4
  [xSM4_B_Enable] -> Merge12/5
  [xSM5_B_Enable] -> Merge12/6
  [xSM6_B_Enable] -> Merge12/7
  [xSM7_B_Enable] -> Merge12/8
  Merge12/1 -> [xTmComprCtrl_B_Enable]  "xTmComprCtrl_B_Enable"

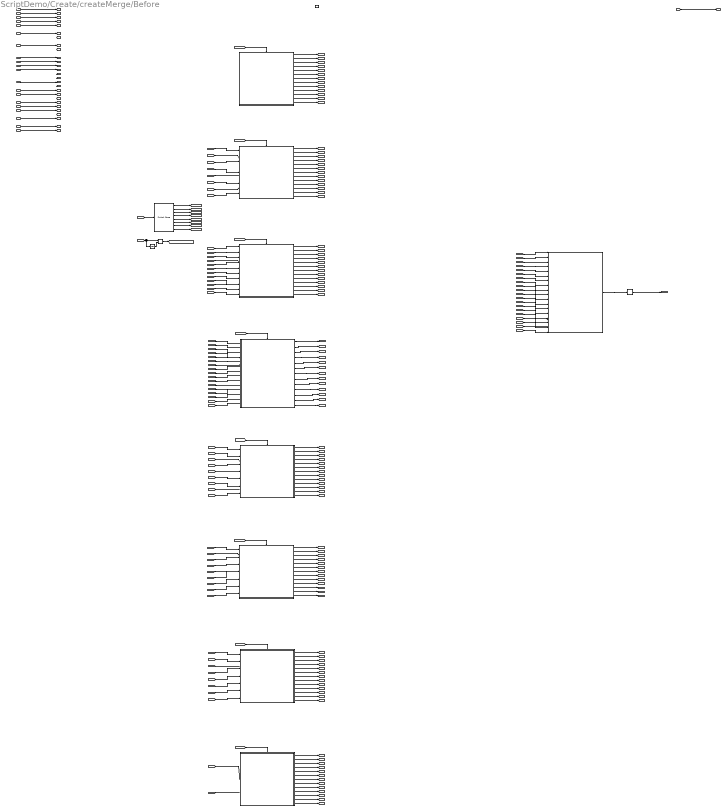
== system ScriptDemo/Create/createMerge/Before ==
  sTmComprCtrl_D_u8HvacFlowLevel : Inport  OutDataTypeStr=uint8
  sTmSigProces_Te_s32EvapFanReqRamp : Inport  Port=2  OutDataTypeStr=single
  sTmDiag_D_u8TeEvapFltSt : Inport  Port=3  OutDataTypeStr=uint8
  sTmIn_D_u8DCChrgSt : Inport  Port=4  OutDataTypeStr=uint8
  sTmIn_D_u8HeatPump : Inport  Port=5  OutDataTypeStr=uint8
  sTmIn_Te_s32BattHv : Inport  Port=6  OutDataTypeStr=single
  sTmIn_X_s32ClimtRcirc : Inport  Port=7  OutDataTypeStr=single
  sTmSigProces_D_u8BattThermReq : Inport  Port=8  OutDataTypeStr=uint8
  sTmSigProces_D_u8HvBattCoolgReq : Inport  Port=9  OutDataTypeStr=uint8
  sTmSigProces_Te_s32EvapFanFilter : Inport  Port=10  OutDataTypeStr=single
  sTmSigProces_Te_s32HeatrAirTReqRamp : Inport  Port=11  OutDataTypeStr=single
  sTmSigProces_Te_s32HvacHexAirTFilter : Inport  Port=12  OutDataTypeStr=single
  sTmSigProces_Te_s32SatHp : Inport  Port=13  OutDataTypeStr=single
  sTmSigProces_Te_s32SatLp : Inport  Port=14  OutDataTypeStr=single
  xTmComprCtrl_B_CompOnReqCompOn : Inport  Port=15  OutDataTypeStr=boolean
  xTmComprCtrl_B_ReduceRpm : Inport  Port=16  OutDataTypeStr=boolean
  yTmHvchCtrl_B_HpcPtcEnad : Inport  Port=17  OutDataTypeStr=boolean
  yTmRefriModeMgr_B_CoolOCRMode : Inport  Port=18  OutDataTypeStr=boolean
  sTmSigProces_Pw_i16ReqPwrForCool : Inport  Port=19  OutDataTypeStr=int16
  yTmRefriModeMgr_B_HeatModeInCycle : Inport  Port=20  OutDataTypeStr=boolean
  Enable : EnablePort
  ID29332_RpmPI : Subsystem
  Relational Operator : RelationalOperator  Operator=~=  OutDataTypeStr=boolean  RndMeth=Simplest  InputSameDT=off
  SM0 : Subsystem
  SM1SM21 : Subsystem
  SM2SM22 : Subsystem
  SM3SM23 : Subsystem
  SM4 : Subsystem
  SM5 : Subsystem
  SM6 : Subsystem
  SM7 : Subsystem
  Signal Conversion : SignalConversion  OverrideOpt=off
  Switch Case : SwitchCase  CaseConditions={0,[1,21],[2,22],[3,23],4,5,6,7}  ShowDefaultCase=off
  Unit Delay : UnitDelay  SampleTime=-1  HasFrameUpgradeWarning=on
  sTmComprCtrl_n_u16CompRpmReqNorm : Outport  OutDataTypeStr=uint16
  wires:
  [yTmRefriModeMgr_B_CoolOCRMode] -> SM2SM22/9(yTmRefriModeMgr_B_CoolOCRMode)
  ? -> [sTmIn_Te_s32HvBattCooltTReq]
  [sTmSigProces_D_u8BattThermReq] -> SM3SM23/8(sTmSigProces_D_u8BattThermReq)
  [sTmSigProces_Te_s32TempInlet] -> ?
  ? -> [yTmRefriModeMgr_B_CoolModeInCycle]
  [sTmSigProces_Te_s32SatHp] -> SM5/4(sTmSigProces_Te_s32SatHp)
  [sTmRefriModeMgr_D_u8HPCurMode] -> ?
  [yTmRefriModeMgr_B_HeatModeInCycle] -> SM4/7(yTmRefriModeMgr_B_HeatModeInCycle)
  [xTmComprCtrl_B_ModeChanged] -> SM3SM23/13(xTmComprCtrl_B_ModeChanged)
  [yTmRefriModeMgr_B_HeatModeInCycle] -> SM6/7(yTmRefriModeMgr_B_HeatModeInCycle)
  [yTmRefriModeMgr_B_CoolModeInCycle] -> ?
  [SM5] -> SM5/Action
  sTmSigProces_Te_s32SatLp/1 -> [sTmSigProces_Te_s32SatLp]
  sTmIn_X_s32ClimtRcirc/1 -> [sTmIn_X_s32ClimtRcirc]
  yTmRefriModeMgr_B_HeatModeInCycle/1 -> [yTmRefriModeMgr_B_HeatModeInCycle]
  yTmRefriModeMgr_B_CoolOCRMode/1 -> [yTmRefriModeMgr_B_CoolOCRMode]
  [yTmRefriModeMgr_B_HeatModeInCycle] -> ID29332_RpmPI/18(yTmRefriModeMgr_B_HeatModeInCycle)
  yTmHvchCtrl_B_HpcPtcEnad/1 -> [yTmHvchCtrl_B_HpcPtcEnad]
  [sTmSigProces_Te_s32EvapFanFilter] -> ID29332_RpmPI/17(sTmSigProces_Te_s32EvapFanFilter)
  [sTmSigProces_D_u8HvBattCoolgReq] -> SM3SM23/9(sTmSigProces_D_u8HvBattCoolgReq)
  [sTmSigProces_Te_s32HvacHexAirTFilter] -> SM5/3(sTmSigProces_Te_s32HvacHexAirTFilter)
  ? -> [sTmSigProces_Te_s32HvBattCooltTFilter]
  [yTmRefriModeMgr_B_CoolOCRMode] -> SM3SM23/14(yTmRefriModeMgr_B_CoolOCRMode)
  [yTmHvchCtrl_B_HpcPtcEnad] -> SM5/7(yTmHvchCtrl_B_HpcPtcEnad)
  [sTmComprCtrl_D_u8HvacFlowLevel] -> SM5/5(sTmComprCtrl_D_u8HvacFlowLevel)
  sTmSigProces_D_u8HvBattCoolgReq/1 -> [sTmSigProces_D_u8HvBattCoolgReq]
  [xTmComprCtrl_B_ReduceRpm] -> ID29332_RpmPI/16(xTmComprCtrl_B_ReduceRpm)
  ? -> [sTmSigProces_Te_s32HvBattCooltTOutFilter]
  sTmSigProces_Pw_i16ReqPwrForCool/1 -> [sTmSigProces_Pw_i16ReqPwrForCool]
  [sTmSigProces_Te_s32TAmb] -> ?
  [sTmIn_Te_s32BattHv] -> SM3SM23/5(sTmIn_Te_s32BattHv)
  [sTmComprCtrl_D_u8HvacFlowLevel] -> SM6/4(sTmComprCtrl_D_u8HvacFlowLevel)
  Switch Case/7 -> [SM6]
  Switch Case/5 -> [SM4]
  ? -> [sTmSigProces_Te_s32TempInlet]
  [xTmComprCtrl_B_CompOnReqCompOn] -> SM5/6(xTmComprCtrl_B_CompOnReqCompOn)
  [rTmComprCtrl_n_u16ComprRpmKp] -> ID29332_RpmPI/6(rTmComprCtrl_n_u16ComprRpmKp)
  [SM0] -> SM0/Action
  xTmComprCtrl_B_ReduceRpm/1 -> [xTmComprCtrl_B_ReduceRpm]
  [sTmSigProces_Te_s32HeatrAirTReqRamp] -> SM6/1(sTmSigProces_Te_s32HeatrAirTReqRamp)
  Relational Operator/1 -> [xTmComprCtrl_B_ModeChanged]
  [xTmComprCtrl_B_CompOnReqCompOn] -> SM3SM23/12(xTmComprCtrl_B_CompOnReqCompOn)
  sTmSigProces_Te_s32EvapFanFilter/1 -> [sTmSigProces_Te_s32EvapFanFilter]
  [xTmComprCtrl_B_CompOnReqCompOn] -> SM6/5(xTmComprCtrl_B_CompOnReqCompOn)
  [sTmSigProces_Te_s32HvacHexAirTFilter] -> SM4/2(sTmSigProces_Te_s32HvacHexAirTFilter)
  [sTmSigProces_Te_s32HvBattCooltTFilter] -> ?
  [yTmHvchCtrl_B_HpcPtcEnad] -> SM6/6(yTmHvchCtrl_B_HpcPtcEnad)
  [rTmComprCtrl_Te_s32TempError] -> ID29332_RpmPI/2(rTmComprCtrl_Te_s32TempError)
  [sTmSigProces_Te_s32SatHp] -> SM6/3(sTmSigProces_Te_s32SatHp)
  [sTmIn_D_u8DCChrgSt] -> SM1SM21/1(sTmIn_D_u8DCChrgSt)
  [SM6] -> SM6/Action
  [sTmIn_D_u8DCChrgSt] -> SM3SM23/3(sTmIn_D_u8DCChrgSt)
  [xTmComprCtrl_B_CompOnReqCompOn] -> SM4/5(xTmComprCtrl_B_CompOnReqCompOn)
  [sTmSigProces_Te_s32HvBattCooltTFilter] -> ?
  Switch Case/4 -> [SM3_SM23]
  [rTmComprCtrl_n_u16ComprRpmFF] -> ID29332_RpmPI/4(rTmComprCtrl_n_u16ComprRpmFF)
  [xTmComprCtrl_B_Enable] -> ID29332_RpmPI/14(xTmComprCtrl_B_Enable)
  [sTmSigProces_Te_s32TAmb] -> ?
  [rTmComprCtrl_n_i16KpLowLimit] -> ID29332_RpmPI/10(rTmComprCtrl_n_i16KpLowLimit)
  [rTmComprCtrl_n_u16DisOverrideValue] -> ID29332_RpmPI/7(rTmComprCtrl_n_u16DisOverrideValue)
  xTmComprCtrl_B_CompOnReqCompOn/1 -> [xTmComprCtrl_B_CompOnReqCompOn]
  [rTmComprCtrl_n_u16ComprRpmKi] -> ID29332_RpmPI/5(rTmComprCtrl_n_u16ComprRpmKi)
  [rTmComprCtrl_n_i16KiLowLimit] -> ID29332_RpmPI/8(rTmComprCtrl_n_i16KiLowLimit)
  [xTmComprCtrl_B_ModeChanged] -> ID29332_RpmPI/15(xTmComprCtrl_B_ModeChanged)
  [sTmSigProces_Te_s32HvBattCooltTFilter] -> ?
  [sTmSigProces_Te_s32TempInlet] -> ?
  [sTmIn_Te_s32HvBattCooltTReq] -> ?
  Unit Delay/1 -> Relational Operator/2
  [SM2_SM22] -> SM2SM22/Action
  [sTmIn_D_u8HeatPump] -> SM3SM23/4(sTmIn_D_u8HeatPump)
  [sTmSigProces_Te_s32TAmb] -> ?
  [sTmRefriModeMgr_D_u8HPCurMode] -> Switch Case/1
  [sTmSigProces_Te_s32HeatrAirTReqRamp] -> SM5/2(sTmSigProces_Te_s32HeatrAirTReqRamp)
  [rTmComprCtrl_n_i16KpUpLimit] -> ID29332_RpmPI/11(rTmComprCtrl_n_i16KpUpLimit)
  [sTmComprCtrl_D_u8HvacFlowLevel] -> SM3SM23/7(sTmComprCtrl_D_u8HvacFlowLevel)
  [rTmComprCtrl_Te_s32LowErrStop] -> ID29332_RpmPI/1(rTmComprCtrl_Te_s32LowErrStop)
  [sTmSigProces_Te_s32EvapFanReqRamp] -> SM3SM23/1(sTmSigProces_Te_s32EvapFanReqRamp)
  [sTmSigProces_D_u8HvBattCoolgReq] -> SM1SM21/3(sTmSigProces_D_u8HvBattCoolgReq)
  [sTmComprCtrl_D_u8HvacFlowLevel] -> SM2SM22/5(sTmComprCtrl_D_u8HvacFlowLevel)
  Switch Case/8 -> [SM7]
  [sTmSigProces_Te_s32EvapFanReqRamp] -> SM2SM22/1(sTmSigProces_Te_s32EvapFanReqRamp)
  [sTmRefriModeMgr_D_u8HPCurMode] -> Unit Delay/1, Relational Operator/1
  [SM4] -> SM4/Action
  [sTmSigProces_Te_s32SatLp] -> SM2SM22/7(sTmSigProces_Te_s32SatLp)
  [sTmIn_D_u8HeatPump] -> SM2SM22/3(sTmIn_D_u8HeatPump)
  [sTmSigProces_Te_s32SatLp] -> SM3SM23/11(sTmSigProces_Te_s32SatLp)
  [sTmSigProces_Te_s32EvapFanFilter] -> SM2SM22/6(sTmSigProces_Te_s32EvapFanFilter)
  [sTmSigProces_Te_s32SatHp] -> SM4/3(sTmSigProces_Te_s32SatHp)
  [sTmSigProces_Pw_i16ReqPwrForCool] -> SM2SM22/10(sTmSigProces_Pw_i16ReqPwrForCool)
  [SM7] -> SM7/Action
  ? -> [sTmSigProces_Te_s32TAmb]
  [sTmSigProces_Te_s32TempInlet] -> ?
  [sTmDiag_D_u8TeEvapFltSt] -> SM3SM23/2(sTmDiag_D_u8TeEvapFltSt)
  [sTmSigProces_Te_s32HvacHexAirTFilter] -> SM6/2(sTmSigProces_Te_s32HvacHexAirTFilter)
  [sTmSigProces_Te_s32TAmb] -> ?
  [sTmIn_D_u8HeatPump] -> SM1SM21/5(sTmIn_D_u8HeatPump)
  [yTmRefriModeMgr_B_CoolModeInCycle] -> ?
  [sTmIn_X_s32ClimtRcirc] -> SM2SM22/4(sTmIn_X_s32ClimtRcirc)
  [SM1_SM21] -> SM1SM21/Action
  [sTmIn_X_s32ClimtRcirc] -> SM3SM23/6(sTmIn_X_s32ClimtRcirc)
  [sRpmPI_n_u16CompRpmReq] -> sTmComprCtrl_n_u16CompRpmReqNorm/1
  [sTmSigProces_Te_s32EvapFanFilter] -> SM3SM23/10(sTmSigProces_Te_s32EvapFanFilter)
  Signal Conversion/1 -> [sRpmPI_n_u16CompRpmReq]
  [sTmSigProces_Te_s32TAmb] -> ?
  [sTmDiag_D_u8TeEvapFltSt] -> SM2SM22/2(sTmDiag_D_u8TeEvapFltSt)
  sTmSigProces_Te_s32HeatrAirTReqRamp/1 -> [sTmSigProces_Te_s32HeatrAirTReqRamp]
  [xTmComprCtrl_B_CompOnReqCompOn] -> ID29332_RpmPI/13(xTmComprCtrl_B_CompOnReqCompOn)
  sTmComprCtrl_D_u8HvacFlowLevel/1 -> [sTmComprCtrl_D_u8HvacFlowLevel]
  [sTmSigProces_Te_s32HvBattCooltTOutFilter] -> ?
  sTmDiag_D_u8TeEvapFltSt/1 -> [sTmDiag_D_u8TeEvapFltSt]
  sTmSigProces_Te_s32SatHp/1 -> [sTmSigProces_Te_s32SatHp]
  ? -> [sTmRefriModeMgr_D_u8HPCurMode]
  [xTmComprCtrl_B_CompOnReqCompOn] -> SM1SM21/4(xTmComprCtrl_B_CompOnReqCompOn)
  sTmIn_D_u8DCChrgSt/1 -> [sTmIn_D_u8DCChrgSt]
  [yTmHvchCtrl_B_HpcPtcEnad] -> SM4/6(yTmHvchCtrl_B_HpcPtcEnad)
  [sTmComprCtrl_D_u8HvacFlowLevel] -> SM4/4(sTmComprCtrl_D_u8HvacFlowLevel)
  [sTmIn_Te_s32HvBattCooltTReq] -> ?
  sTmSigProces_Te_s32EvapFanReqRamp/1 -> [sTmSigProces_Te_s32EvapFanReqRamp]
  Switch Case/6 -> [SM5]
  sTmSigProces_Te_s32HvacHexAirTFilter/1 -> [sTmSigProces_Te_s32HvacHexAirTFilter]
  [sTmSigProces_Te_s32SatLp] -> SM5/1(sTmSigProces_Te_s32SatLp)
  Switch Case/3 -> [SM2_SM22]
  ID29332_RpmPI/1(rTmComprCtrl_n_u16CompRpmReqPI) -> Signal Conversion/1  "rTmComprCtrl_n_u16CompRpmReqPI"
  [sTmSigProces_Te_s32HeatrAirTReqRamp] -> SM4/1(sTmSigProces_Te_s32HeatrAirTReqRamp)
  [SM3_SM23] -> SM3SM23/Action
  sTmIn_D_u8HeatPump/1 -> [sTmIn_D_u8HeatPump]
  sTmSigProces_D_u8BattThermReq/1 -> [sTmSigProces_D_u8BattThermReq]
  [rTmComprCtrl_t_u16PIPeriod] -> ID29332_RpmPI/12(rTmComprCtrl_t_u16PIPeriod)
  [sTmSigProces_D_u8BattThermReq] -> SM1SM21/2(sTmSigProces_D_u8BattThermReq)
  Switch Case/2 -> [SM1_SM21]
  Switch Case/1 -> [SM0]
  [rTmComprCtrl_Te_s32UpErrStop] -> ID29332_RpmPI/3(rTmComprCtrl_Te_s32UpErrStop)
  [xTmComprCtrl_B_CompOnReqCompOn] -> SM2SM22/8(xTmComprCtrl_B_CompOnReqCompOn)
  sTmIn_Te_s32BattHv/1 -> [sTmIn_Te_s32BattHv]
  [rTmComprCtrl_n_i16KiUpLimit] -> ID29332_RpmPI/9(rTmComprCtrl_n_i16KiUpLimit)
  SM7/1(rSM7_n_u16DisOverrideValue) -> [rSM7_n_u16DisOverrideValue]
  SM7/2(rSM7_t_u16PIPeriod) -> [rSM7_t_u16PIPeriod]
  SM7/3(xSM7_B_Enable) -> [xSM7_B_Enable]
  SM7/4(rSM7_n_i16KiUpLimit) -> [rSM7_n_i16KiUpLimit]
  SM7/5(rSM7_n_i16KiLowLimit) -> [rSM7_n_i16KiLowLimit]
  SM7/6(rSM7_Te_s32TempError) -> [rSM7_Te_s32TempError]
  SM7/7(rSM7_n_u16ComprRpmFF) -> [rSM7_n_u16ComprRpmFF]
  SM7/8(rSM7_n_u16ComprRpmKp) -> [rSM7_n_u16ComprRpmKp]
  SM7/9(rSM7_n_u16ComprRpmKi) -> [rSM7_n_u16ComprRpmKi]
  SM7/10(rSM7_Te_s32UpErrStop) -> [rSM7_Te_s32UpErrStop]
  SM7/11(rSM7_Te_s32LowErrStop) -> [rSM7_Te_s32LowErrStop]
  SM7/12(rSM7_n_i16KpUpLimit) -> [rSM7_n_i16KpUpLimit]
  SM7/13(rSM7_n_i16KpLowLimit) -> [rSM7_n_i16KpLowLimit]
  SM3SM23/1(rSM3SM23_n_u16ComprRpmKi) -> [rSM3SM23_n_u16ComprRpmKi]
  SM3SM23/2(rSM3SM23_Te_s32UpErrStop) -> [rSM3SM23_Te_s32UpErrStop]
  SM3SM23/3(rSM3SM23_n_u16ComprRpmFF) -> [rSM3SM23_n_u16ComprRpmFF]
  SM3SM23/4(rSM3SM23_n_u16DisOverrideValue) -> [rSM3SM23_n_u16DisOverrideValue]
  SM3SM23/5(rSM3SM23_t_u16PIPeriod) -> [rSM3SM23_t_u16PIPeriod]
  SM3SM23/6(xSM3SM23_B_Enable) -> [xSM3SM23_B_Enable]
  SM3SM23/7(rSM3SM23_n_u16ComprRpmKp) -> [rSM3SM23_n_u16ComprRpmKp]
  SM3SM23/8(rSM3SM23_Te_s32LowErrStop) -> [rSM3SM23_Te_s32LowErrStop]
  SM3SM23/9(rSM3SM23_n_i16KpUpLimit) -> [rSM3SM23_n_i16KpUpLimit]
  SM3SM23/10(rSM3SM23_n_i16KpLowLimit) -> [rSM3SM23_n_i16KpLowLimit]
  SM3SM23/11(rSM3SM23_n_i16KiUpLimit) -> [rSM3SM23_n_i16KiUpLimit]
  SM3SM23/12(rSM3SM23_n_i16KiLowLimit) -> [rSM3SM23_n_i16KiLowLimit]
  SM3SM23/13(rSM3SM23_Te_s32TempError) -> [rSM3SM23_Te_s32TempError]
  SM0/1(rSM0_Te_s32TempError) -> [rSM0_Te_s32TempError]
  SM0/2(rSM0_n_u16ComprRpmFF) -> [rSM0_n_u16ComprRpmFF]
  SM0/3(rSM0_n_u16DisOverrideValue) -> [rSM0_n_u16DisOverrideValue]
  SM0/4(rSM0_t_u16PIPeriod) -> [rSM0_t_u16PIPeriod]
  SM0/5(xSM0_B_Enable) -> [xSM0_B_Enable]
  SM0/6(rSM0_n_u16ComprRpmKp) -> [rSM0_n_u16ComprRpmKp]
  SM0/7(rSM0_n_u16ComprRpmKi) -> [rSM0_n_u16ComprRpmKi]
  SM0/8(rSM0_Te_s32UpErrStop) -> [rSM0_Te_s32UpErrStop]
  SM0/9(rSM0_Te_s32LowErrStop) -> [rSM0_Te_s32LowErrStop]
  SM0/10(rSM0_n_i16KpUpLimit) -> [rSM0_n_i16KpUpLimit]
  SM0/11(rSM0_n_i16KpLowLimit) -> [rSM0_n_i16KpLowLimit]
  SM0/12(rSM0_n_i16KiUpLimit) -> [rSM0_n_i16KiUpLimit]
  SM0/13(rSM0_n_i16KiLowLimit) -> [rSM0_n_i16KiLowLimit]
  SM1SM21/1(rSM1SM21_n_u16DisOverrideValue) -> [rSM1SM21_n_u16DisOverrideValue]
  SM1SM21/2(rSM1SM21_t_u16PIPeriod) -> [rSM1SM21_t_u16PIPeriod]
  SM1SM21/3(rSM1SM21_Te_s32UpErrStop) -> [rSM1SM21_Te_s32UpErrStop]
  SM1SM21/4(rSM1SM21_Te_s32LowErrStop) -> [rSM1SM21_Te_s32LowErrStop]
  SM1SM21/5(rSM1SM21_n_i16KpUpLimit) -> [rSM1SM21_n_i16KpUpLimit]
  SM1SM21/6(rSM1SM21_n_u16ComprRpmFF) -> [rSM1SM21_n_u16ComprRpmFF]
  SM1SM21/7(rSM1SM21_n_u16ComprRpmKp) -> [rSM1SM21_n_u16ComprRpmKp]
  SM1SM21/8(rSM1SM21_n_u16ComprRpmKi) -> [rSM1SM21_n_u16ComprRpmKi]
  SM1SM21/9(rSM1SM21_n_i16KpLowLimit) -> [rSM1SM21_n_i16KpLowLimit]
  SM1SM21/10(rSM1SM21_n_i16KiUpLimit) -> [rSM1SM21_n_i16KiUpLimit]
  SM1SM21/11(rSM1SM21_n_i16KiLowLimit) -> [rSM1SM21_n_i16KiLowLimit]
  SM1SM21/12(xSM1SM21_B_Enable) -> [xSM1SM21_B_Enable]
  SM1SM21/13(rSM1SM21_Te_s32TempError) -> [rSM1SM21_Te_s32TempError]
  SM2SM22/1(rSM2SM22_n_u16DisOverrideValue) -> [rSM2SM22_n_u16DisOverrideValue]
  SM2SM22/2(rSM2SM22_t_u16PIPeriod) -> [rSM2SM22_t_u16PIPeriod]
  SM2SM22/3(rSM2SM22_Te_s32UpErrStop) -> [rSM2SM22_Te_s32UpErrStop]
  SM2SM22/4(rSM2SM22_n_u16ComprRpmFF) -> [rSM2SM22_n_u16ComprRpmFF]
  SM2SM22/5(rSM2SM22_n_u16ComprRpmKp) -> [rSM2SM22_n_u16ComprRpmKp]
  SM2SM22/6(rSM2SM22_n_u16ComprRpmKi) -> [rSM2SM22_n_u16ComprRpmKi]
  SM2SM22/7(rSM2SM22_Te_s32LowErrStop) -> [rSM2SM22_Te_s32LowErrStop]
  SM2SM22/8(rSM2SM22_n_i16KpUpLimit) -> [rSM2SM22_n_i16KpUpLimit]
  SM2SM22/9(rSM2SM22_n_i16KpLowLimit) -> [rSM2SM22_n_i16KpLowLimit]
  SM2SM22/10(rSM2SM22_n_i16KiUpLimit) -> [rSM2SM22_n_i16KiUpLimit]
  SM2SM22/11(rSM2SM22_n_i16KiLowLimit) -> [rSM2SM22_n_i16KiLowLimit]
  SM2SM22/12(xSM2SM22_B_Enable) -> [xSM2SM22_B_Enable]
  SM2SM22/13(rSM2SM22_Te_s32TempError) -> [rSM2SM22_Te_s32TempError]
  SM4/1(rSM4_n_u16DisOverrideValue) -> [rSM4_n_u16DisOverrideValue]
  SM4/2(rSM4_t_u16PIPeriod) -> [rSM4_t_u16PIPeriod]
  SM4/3(rSM4_Te_s32UpErrStop) -> [rSM4_Te_s32UpErrStop]
  SM4/4(rSM4_n_u16ComprRpmFF) -> [rSM4_n_u16ComprRpmFF]
  SM4/5(rSM4_n_u16ComprRpmKp) -> [rSM4_n_u16ComprRpmKp]
  SM4/6(rSM4_Te_s32LowErrStop) -> [rSM4_Te_s32LowErrStop]
  SM4/7(rSM4_n_i16KpUpLimit) -> [rSM4_n_i16KpUpLimit]
  SM4/8(rSM4_n_i16KpLowLimit) -> [rSM4_n_i16KpLowLimit]
  SM4/9(rSM4_n_i16KiUpLimit) -> [rSM4_n_i16KiUpLimit]
  SM4/10(rSM4_n_i16KiLowLimit) -> [rSM4_n_i16KiLowLimit]
  SM4/11(xSM4_B_Enable) -> [xSM4_B_Enable]
  SM4/12(rSM4_n_u16ComprRpmKi) -> [rSM4_n_u16ComprRpmKi]
  SM4/13(rSM4_Te_s32TempError) -> [rSM4_Te_s32TempError]
  SM5/1(rSM5_n_u16DisOverrideValue) -> [rSM5_n_u16DisOverrideValue]
  SM5/2(rSM5_t_u16PIPeriod) -> [rSM5_t_u16PIPeriod]
  SM5/3(rSM5_Te_s32UpErrStop) -> [rSM5_Te_s32UpErrStop]
  SM5/4(rSM5_n_u16ComprRpmFF) -> [rSM5_n_u16ComprRpmFF]
  SM5/5(rSM5_n_u16ComprRpmKp) -> [rSM5_n_u16ComprRpmKp]
  SM5/6(rSM5_Te_s32LowErrStop) -> [rSM5_Te_s32LowErrStop]
  SM5/7(rSM5_n_i16KpUpLimit) -> [rSM5_n_i16KpUpLimit]
  SM5/8(rSM5_n_i16KpLowLimit) -> [rSM5_n_i16KpLowLimit]
  SM5/9(rSM5_n_i16KiUpLimit) -> [rSM5_n_i16KiUpLimit]
  SM5/10(rSM5_n_i16KiLowLimit) -> [rSM5_n_i16KiLowLimit]
  SM5/11(xSM5_B_Enable) -> [xSM5_B_Enable]
  SM5/12(rSM5_n_u16ComprRpmKi) -> [rSM5_n_u16ComprRpmKi]
  SM5/13(rSM5_Te_s32TempError) -> [rSM5_Te_s32TempError]
  SM6/1(rSM6_n_u16DisOverrideValue) -> [rSM6_n_u16DisOverrideValue]
  SM6/2(rSM6_t_u16PIPeriod) -> [rSM6_t_u16PIPeriod]
  SM6/3(rSM6_Te_s32UpErrStop) -> [rSM6_Te_s32UpErrStop]
  SM6/4(rSM6_n_u16ComprRpmFF) -> [rSM6_n_u16ComprRpmFF]
  SM6/5(rSM6_n_u16ComprRpmKp) -> [rSM6_n_u16ComprRpmKp]
  SM6/6(rSM6_Te_s32LowErrStop) -> [rSM6_Te_s32LowErrStop]
  SM6/7(rSM6_n_i16KpUpLimit) -> [rSM6_n_i16KpUpLimit]
  SM6/8(rSM6_n_i16KpLowLimit) -> [rSM6_n_i16KpLowLimit]
  SM6/9(rSM6_n_i16KiUpLimit) -> [rSM6_n_i16KiUpLimit]
  SM6/10(rSM6_n_i16KiLowLimit) -> [rSM6_n_i16KiLowLimit]
  SM6/11(xSM6_B_Enable) -> [xSM6_B_Enable]
  SM6/12(rSM6_n_u16ComprRpmKi) -> [rSM6_n_u16ComprRpmKi]
  SM6/13(rSM6_Te_s32TempError) -> [rSM6_Te_s32TempError]

== system ScriptDemo/Create/createPorts/createPorts ==
  After : Subsystem

== system ScriptDemo/Create/createPorts/createPortsGoto ==
  note: %% 输入参数处理
      | p = inputParser; % 函数的输入解析器
      | addParameter(p, 'posIn' ,[-500 0]); % 输入端口位置
      | addParameter(p, 'posOut' ,[500 0]); % 输出端口位置
      | addParameter(p, 'step' ,30); % 端口间隔
      | addParameter(p, 'gotoLength' ,180); % goto from 的宽度
      | addParameter(p, 'inList' ,{}); % 根据如果指定了inList列表，则会根据此列表进行创建输入端口及goto
      | addParameter(p, 'outList' ,{}); % 根据如果指定了outList列表，则会根据此列表进行创建输出端口及from
      | addParameter(p, 'NAStr' , 'NA' ); % 列表中忽略的字段，比如遇到'NA'，则会跳过此信号
      | addParameter(p, 'mode' , 'keep' ); % 可选：pre, tail, keep
      | addParameter(p, 'template' , 'Template' ); % 模板名称
      | addParameter(p, 'sheet' , 'Signals' ); % 模板工作表
      | addParameter(p, 'inRecognName' , 'Input' ); % 输入信号识别字段，位于PortType列
      | addParameter(p, 'outRecognName' , 'Output' ); % 输出信号识别字段，位于PortType列
  After1 : Subsystem
  After2 : Subsystem
  After3 : Subsystem

== system ScriptDemo/Create/createPorts/createPortsGotoUpdate ==
  After : Subsystem
  After1 : Subsystem
  Before : Subsystem
  wires:
  [sTmIn_Pw_s32HvCoolgAllwd] -> After/1(sTmIn_Pw_s32HvCoolgAllwd)
  [xTmComprCtrl_B_CompOnReqCompOn] -> After/2(xTmComprCtrl_B_CompOnReqCompOn)
  After/1(sTmComprCtrl_Pw_s32ElacCmprMaxState) -> [sTmComprCtrl_Pw_s32ElacCmprMaxState]
  After/2(yTmComprCtrl_B_HpcCoolgLimd) -> [yTmComprCtrl_B_HpcCoolgLimd]
  [sTmIn_Pw_s32HvCoolgAllwd] -> After1/1(sTmIn_Pw_s32HvCoolgAllwd)
  [xTmComprCtrl_B_CompOnReqCompOn] -> After1/2(xTmComprCtrl_B_CompOnReqCompOn)
  After1/1(rAfter1_Pw_s32ElacCmprMaxState) -> [rAfter1_Pw_s32ElacCmprMaxState]
  After1/2(xAfter1_B_HpcCoolgLimd) -> [xAfter1_B_HpcCoolgLimd]

== system ScriptDemo/Create/createPorts/createPortsGotoUpdateLoop ==
  note: % 输入参数处理
      | addParameter(p, 'path' ,gcs); % 当前路径
      | addParameter(p, 'topLev' ,bdroot); % 循环结束的模型层， default is bdroot, or define as 'TmComprCtrl'
      | addParameter(p, 'resoveValue' ,true); % 是否解析信号
  After : Subsystem
  Before : Subsystem
